simulink model "complexEqu"  (R2023b)
settings: Solver=VariableStepAuto  StartTime=0.0  StopTime=10.0  RelTol=1e-3
settings Model: Creator=mhagh  LastModifiedBy=mhagh

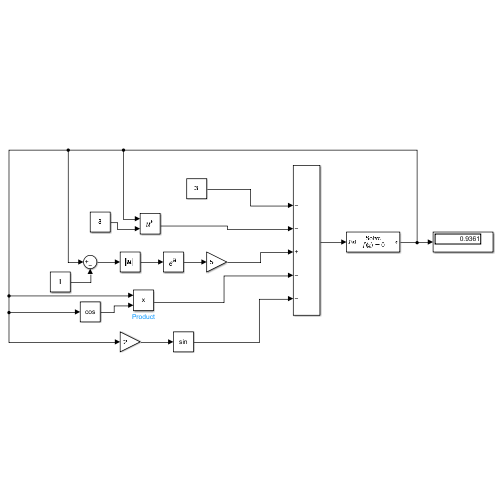
[thumbnail: Simulink's stored preview of the top-level diagram]
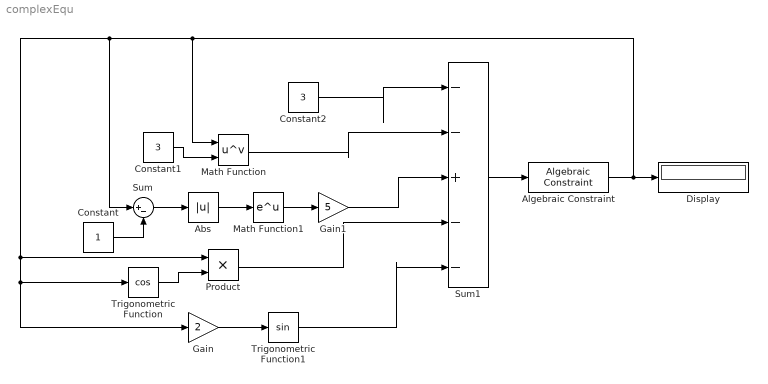
== system complexEqu ==
  Abs : Abs  SaturateOnIntegerOverflow=off
  Algebraic Constraint : AlgebraicConstraint
  Constant : Constant
  Constant1 : Constant  Value=3
  Constant2 : Constant  Value=3
  Display : Display
  Gain : Gain  Gain=2
  Gain1 : Gain  Gain=5
  Math Function : Math  Operator=pow
  Math Function1 : Math
  Product : Product
  Sum : Sum  Inputs=|+-
  Sum1 : Sum  Inputs=|--+--
  Trigonometric Function : Trigonometry  Operator=cos
  Trigonometric Function1 : Trigonometry
  wires:
  Math Function1/1 -> Gain1/1
  Sum1/1 -> Algebraic Constraint/1
  Algebraic Constraint/1 -> Math Function/1, Trigonometric Function/1, Gain/1, Product/1, Sum/1, Display/1
  Constant/1 -> Sum/2
  Constant1/1 -> Math Function/2
  Constant2/1 -> Sum1/1
  Math Function/1 -> Sum1/2
  Sum/1 -> Abs/1
  Abs/1 -> Math Function1/1
  Gain1/1 -> Sum1/3
  Trigonometric Function/1 -> Product/2
  Product/1 -> Sum1/4
  Gain/1 -> Trigonometric Function1/1
  Trigonometric Function1/1 -> Sum1/5
